simulink model "raspberrypi_simple_websocket"  (Simulink 10.0)
settings: Solver=FixedStepDiscrete  StartTime=0.0  StopTime=Inf  FixedStep=0.02  RelTol=1e-3  EnableMultiTasking=on
libraries: raspberrypiNetworklib x2, simulink x1
settings Model: FPTRunName=Active  Creator=The MathWorks, Inc.  LastModifiedBy=kkoichi  EnablePacing=on  ExtModeTrigDuration=2
settings SolverCC: PositivePriorityOrder=on
settings DataIOCC: LimitDataPoints=on  ReturnWorkspaceOutputs=on
settings OptimizationCC: ExpressionDepthLimit=2147483647  LifeSpan=Inf  MaxStackSize=64
settings DebuggingCC: SaveWithDisabledLinksMsg=none  SaveWithParameterizedLinksMsg=none  FcnCallInpInsideContextMsg=warning  AllowSymbolicDim=off  StateNameClashWarn=warning
settings HardwareCC: ProdLargestAtomicInteger=Long  ProdLargestAtomicFloat=Double  ProdIntDivRoundTo=Zero  ProdEndianess=LittleEndian  ProdLongLongMode=on  ProdHWDeviceType=ARM Compatible->ARM Cortex  UseEmbeddedCoderFeatures=off  UseSimulinkCoderFeatures=off
settings RTWCC: Description=Embedded Coder  SystemTargetFile=ert.tlc  HardwareBoard=Raspberry Pi  TLCOptions="-aInlineSetEventsForThisBaseRateFcn=TLC_FALSE -aSuppressMultiTaskScheduler=TLC_FALSE  -aRateBasedStepFcn=0"  TemplateMakefile=ert_default_tmf  GenerateReport=on  RTWVerbose=off  Toolchain=GNU GCC Embedded Linux  BuildConfiguration=Faster Runs  LaunchReport=on
settings MATStruct: className=codertarget.tools.BuildHook  argsTopModelOnly=[]  excludedModels=[]  includeReferencedModels=on  includeTopModel=on  enabled=on  UseCoderTarget=[1.0]  TargetHardware=Raspberry Pi  RTOS=Linux  RTOSBaseRateTaskPriority=40  DetectTaskOverruns=[0.0]  Scheduler_interrupt_source=[0.0]  DataVersion=2016.02  IOBlocksMode=deployed  IPAddress=codertarget.raspi.getDeviceAddress  Port=17725  Verbose=[0.0]  RunInBackground=[0.0]  Configuration=XCP on TCP/IP  signalBufferSize=[1000000.0]  DeviceAddress=192.168.8.114  Username=pi  Password=raspberry  BuildDir=/home/pi  SerialNumber=172.19.74.109  OnlineBuildDir=/home/pi  BuildAction=Build and run  RunOnBoot=[0.0]  SPI0CE0BusSpeed=500  SPI0CE1BusSpeed=500  CANBusSpeed=500  CANOscillatorFrequency=16  InterruptPin=12  AllowAllFilter=[1.0]  Buffer0IDType=Normal  AcceptanceMask0=0  AcceptanceFilter0=255  AcceptanceFilter1=255  Buffer1IDType=Normal  AcceptanceMask1=0  AcceptanceFilter2=255  AcceptanceFilter3=255  AcceptanceFilter4=255  AcceptanceFilter5=255  InverseFilter0=[0.0]  InverseFilter1=[0.0]  Buffer2IDType=Extended  AcceptanceMask2=0  InverseFilter2=[0.0]  Buffer3IDType=Extended  AcceptanceMask3=0  InverseFilter3=[0.0]  BrokerAddress=mqtt.thingspeak.com  TransportLayerType=TCP/IP  ModelTransportDataFcn=codertarget.raspi.ioclient.getModelTransportInfo  ServerDeployFcn=codertarget.raspi.ioclient.deployServer  TransportLayerTypeOnline=Internet  Modbus_comms=TCP/IP  Modbus_mode=Master  Modbus_serverRemotePort=502  Modbus_serverLocalPort=502  Modbus_configCoil=1  Modbus_CoilAddr=0  Modbus_CoilNum=1  Modbus_configInput=1  Modbus_InputAddr=0  Modbus_InputNum=1  Modbus_configHoldingReg=1  Modbus_HoldingRegAddr=0  Modbus_HoldingRegNum=1  Modbus_configInputReg=1  Modbus_InputRegAddr=0  Modbus_InputRegNum=1  Modbus_MasterTimeout=100  EnableDeployment=[0.0]  IPAddressType=Device address  WebSocketPort=8000  HTTPPort=8888
settings CodeAppCC: ForceParamTrailComments=on  OperatorAnnotations=on  MATLABSourceComments=on
settings ERTTargetCC: MultiwordLength=2048  ERTCustomFileBanners=off  SupportContinuousTime=on  SupportNonInlinedSFcns=on  RemoveResetFunc=off  SupportVariableSizeSignals=on  ModelStepFunctionPrototypeControlCompliant=off  ExtModeTransport=2  ExtModeStaticAlloc=on  ExtModeMexFile=ext_xcp  ExtModeIntrfLevel=Level2 - Open
settings ConfigComp: CovExternalEMLEnable=off  CovSFcnEnable=off

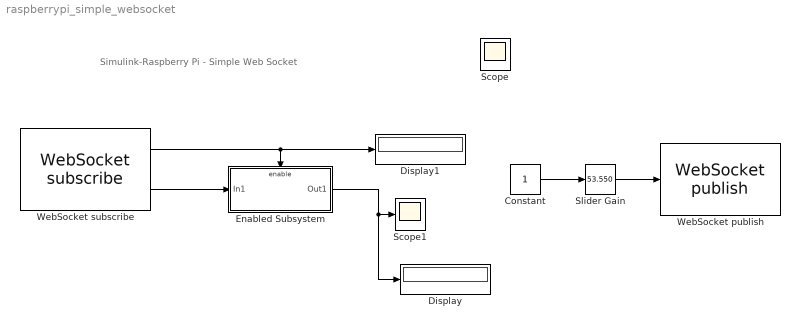
== system raspberrypi_simple_websocket ==
  note: Simulink-Raspberry Pi - Simple Web Socket
  Constant : Constant
  Display : Display
  Display1 : Display
  Enabled Subsystem : Subsystem  TreatAsAtomicUnit=on
  Scope1 : Scope
  Slider Gain : simulink/Math Operations/Slider Gain  gain=53.550  low=0  high=255
  WebSocket publish : raspberrypiNetworklib/WebSocket publish  UniqueBlockID=Test  IPAddress=192.168.8.114  Port=9137  NumberOfSignals=1  webSocketId=raspberrypi_simple_websocket/WebSocket_publish  BlockPlatform=RASPBERRYPI
      settings: SourceProductBaseCode=RASPPI
      settings: AttributesFormatString=|
      | <IPAddress=%<IPAddress>>
      | <Port=%<Port>>
  WebSocket subscribe : raspberrypiNetworklib/WebSocket subscribe  IPAddress=192.168.8.114  Port=9137  OutputCfg=Mask Dialog  numSignals=1  Dsize1=1  Dtype1=double  Dsize2=1  Dtype2=double  Dsize3=1  Dtype3=double  Dsize4=1  Dtype4=double  Dsize5=1  Dtype5=double  Dsize6=1  Dtype6=double  Dsize7=1  Dtype7=double  Dsize8=1  Dtype8=double  Dsize9=1  Dtype9=double  Dsize10=1  Dtype10=double  Sampletime=-1  NumberOfSignals=1  webSocketId=raspberrypi_simple_websocket/WebSocket_subscribe  BlockPlatform=RASPBERRYPI
      settings: SourceProductBaseCode=RASPPI
      settings: AttributesFormatString=|
      | <IPAddress=%<IPAddress>>
      | <Port=%<Port>>
  Scope : Scope
  wires:
  Constant/1 -> Slider Gain/1
  WebSocket subscribe/1 -> Enabled Subsystem/Enable, Display1/1
  Slider Gain/1 -> WebSocket publish/1
  Enabled Subsystem/1(Out1) -> Display/1, Scope1/1
  WebSocket subscribe/2 -> Enabled Subsystem/1(In1)

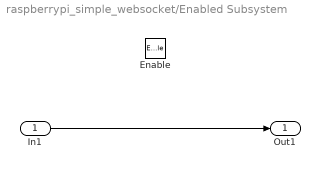
== system raspberrypi_simple_websocket/Enabled Subsystem ==
  In1 : Inport
  Enable : EnablePort
  Out1 : Outport  InitialOutput=90
  wires:
  In1/1 -> Out1/1
